simulink model "bouncing_ball"  (R2018a)
settings: Solver=VariableStepAuto  StartTime=0.0  StopTime=15  RelTol=1e-3
settings Model: Creator=U500304  LastModifiedBy=U500304

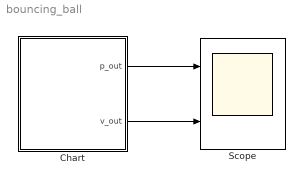
== system bouncing_ball ==
  Chart : Stateflow chart  TreatAsAtomicUnit=on
  Scope : Scope  NumInputPorts=2
  wires:
  Chart/1(p_out) -> Scope/1
  Chart/2(v_out) -> Scope/2

== stateflow chart bouncing_ball/Chart ==
  settings: updateMethod=CONTINUOUS
  state Falling
    du:
    p_dot = v;
    v_dot = -9.81;
    p_out = p;
    v_out = v;
  state Still
  (default) -> Falling : {
      | p = 10;
      | v = 5;
      | }
  Falling -> Falling [order 2] : [p <= 0 && v < 0]
      | {p = 0; v = -0.8 * v;}
  Falling -> Still [order 1] : [p <= 0 && v < 0 && v > -1]
      | {p = 0; v = 0;}
  data: p_out output; v_out output; v local; p local
  data v settings: updateMethod=SF_CONTINUOUS_TIME_DATA
  data p settings: updateMethod=SF_CONTINUOUS_TIME_DATA
